simulink model "cannon_ball"  (R2023a)
settings: Solver=VariableStepAuto  StartTime=0.0  StopTime=10.0  RelTol=1e-3
settings Model: Creator=asd19005  LastModifiedBy=asd19005

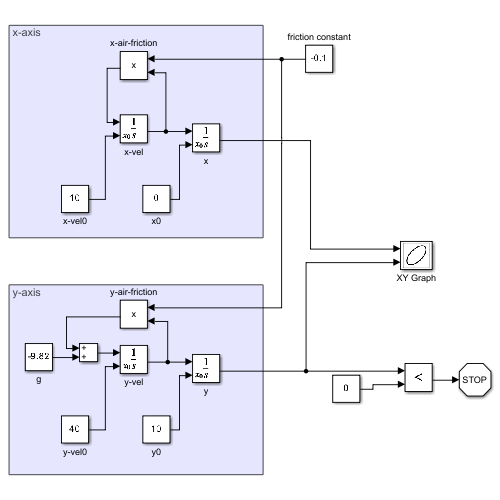
[thumbnail: Simulink's stored preview of the top-level diagram]
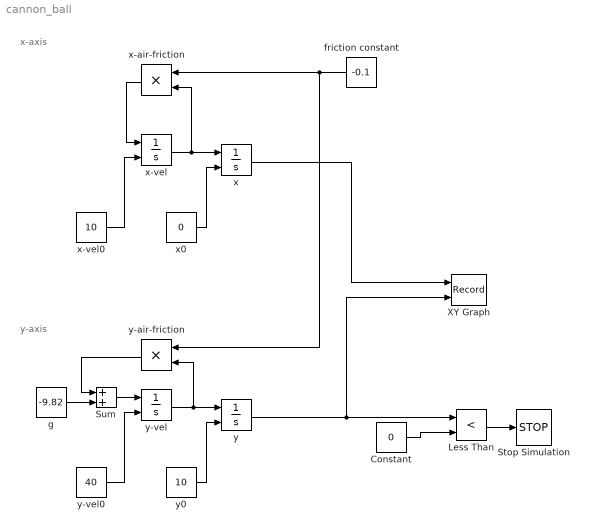
== system cannon_ball ==
  note: x-axis
  note: y-axis
  Constant : Constant  Value=0
  Less Than : RelationalOperator  Operator=<  OutDataTypeStr=boolean  RndMeth=Simplest  InputSameDT=off
  Stop Simulation : Stop
  Sum : Sum
  XY Graph : Record  FileSettingsInternal="{\"entries\":[{\"content\":{\"excelSettings\":{\"content\":{},\"type\":\"Streamout.ExcelSettings\"}},\"type\":\"Streamout.FileSettingStorage\",\"uuid\":\"cf30e1b8-fb18-4b4c-a922-f001dc3dc8db\"}],\"packageUris\":[\"http://schema.mathworks.com/mf0/streamout_blocks/R2020a\"],\"version\":\"1.0\"}"  Layout=[1 1]  SignalsInternal="{\"entries\":[{\"content\":{\"signals\":[{\"content\":{\"blockPath\":[\"cannon_ball/XY Graph\"],\"dimensions\":[1],\"domain\":\"cannon_ball/XY Graph\",\"lineColor\":\"#a2142f\",\"plots\":[1],\"port\":1,\"sid\":[\"\"],\"signalID\":320,\"signalName\":\"x\"},\"type\":\"RecordBlkView.Signal\",\"uuid\":\"7bc2fc54-d4ed-435f-b7a2-032132725fb7\"},{\"content\":{\"blockPath\":[\"cannon_ball/XY Graph\"],\"dimensions\":[1],\"domain\":\"cannon_ball/XY Graph\",\"lineColor\":\"#139fff\",\"plots\":[1],\"port\":2,\"sid\":[\"\"],\"signalID\":324,\"signalName\":\"y\"},\"type\":\"RecordBlkView.Signal\",\"uuid\":\"35534c2a-12c8-4edf-9e6c-0bfdbdcaf6ec\"}]},\"type\":\"RecordBlkView.InputSignals\",\"uuid\":\"39627b1f-027b-49c6-b4f6-8e96554cbea5\"}],\"packageUris\":[\"http://schema.mathworks.com/mf0/streamout_blocks/R2020a\"],\"version\":\"1.0\"}"  VisualizationBindings="{\"xyplotplugin\":{\"info\":[{\"series\":[{\"bindingParametersList\":[{\"parameter\":\"X-Axis\",\"signalID\":320,\"signalName\":\"x\"},{\"parameter\":\"Y-Axis\",\"signalID\":324,\"signalName\":\"y\"}],\"seriesID\":270}],\"subplotID\":1}]}}"  CompatibilityTag=XY
  friction constant : Constant  Value=-0.1
  g : Constant  Value=-9.82
  x : Integrator  InitialConditionSource=external  InitialCondition=100
  x-air-friction : Product
  x-vel : Integrator  InitialConditionSource=external  InitialCondition=10
  x-vel0 : Constant  Value=10
  x0 : Constant  Value=0
  y : Integrator  InitialConditionSource=external  InitialCondition=100
  y-air-friction : Product
  y-vel : Integrator  InitialConditionSource=external  InitialCondition=10
  y-vel0 : Constant  Value=40
  y0 : Constant  Value=10
  wires:
  y-vel/1 -> y-air-friction/2, y/1
  y/1 -> XY Graph/2, Less Than/1
  y0/1 -> y/2
  y-vel0/1 -> y-vel/2
  x-vel/1 -> x-air-friction/2, x/1
  x0/1 -> x/2
  x-vel0/1 -> x-vel/2
  friction constant/1 -> y-air-friction/1, x-air-friction/1
  x-air-friction/1 -> x-vel/1
  x/1 -> XY Graph/1
  y-air-friction/1 -> Sum/1
  g/1 -> Sum/2
  Sum/1 -> y-vel/1
  Less Than/1 -> Stop Simulation/1
  Constant/1 -> Less Than/2
